simulink model "respiratory"  (R2020a)
settings: Solver=VariableStepAuto  StartTime=0.0  StopTime=17.0  RelTol=1e-3
settings Model: Creator=PrasunOrchi  LastModifiedBy=PrasunOrchi

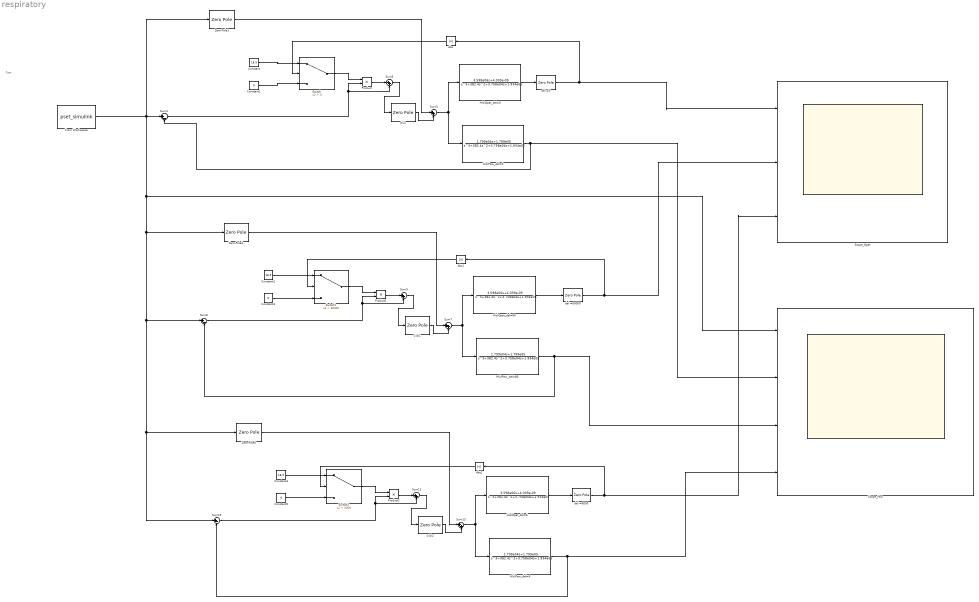
== system respiratory ==
  note: Pset
  Abs : Abs
  Abs1 : Abs
  Abs2 : Abs
  C(s) : ZeroPole  Zeros=[]  Poles=[0]  Gain=[0.4]
  C(s)1 : ZeroPole  Zeros=[]  Poles=[0]  Gain=[0.4]
  C(s)2 : ZeroPole  Zeros=[]  Poles=[0]  Gain=[0.4]
  Constant : Constant  Value=18.5
  Constant1 : Constant  Value=0
  Constant2 : Constant  Value=18.5
  Constant3 : Constant  Value=0
  Constant4 : Constant  Value=18.5
  Constant5 : Constant  Value=0
  From Workspace : FromWorkspace  VariableName=pset_simulink
  H(s)Paw_del=0 : TransferFcn  Numerator=[1.799e04 1.799e05]  Denominator=[1 382.4 3.758e04 1.934e05]
  H(s)Paw_del=6 : TransferFcn  Numerator=[1.799e04 1.799e05]  Denominator=[1 382.4 3.758e04 1.934e05]
  H(s)Paw_del=80 : TransferFcn  Numerator=[1.799e04 1.799e05]  Denominator=[1 382.4 3.758e04 1.934e05]
  H(s)Qpat_del=0 : TransferFcn  Numerator=[3.598e06 4.039e-09]  Denominator=[1 382.4 3.758e04 1.934e05]
  H(s)Qpat_del=6 : TransferFcn  Numerator=[3.598e06 4.039e-09]  Denominator=[1 382.4 3.758e04 1.934e05]
  H(s)Qpat_del=80 : TransferFcn  Numerator=[3.598e06 4.039e-09]  Denominator=[1 382.4 3.758e04 1.934e05]
  Product : Product
  Product1 : Product
  Product2 : Product
  Scope_Paw : Scope  NumInputPorts=4
  Scope_Qpat : Scope  NumInputPorts=3
  Sum10 : Sum  Inputs=|+-
  Sum{3,5,7,9,11,13} (6 alike) : Sum  Inputs=|++
  Sum4 : Sum  Inputs=|+-
  Sum8 : Sum  Inputs=|+-
  Switch : Switch  Criteria=u2 > Threshold
  Switch1 : Switch  Criteria=u2 > Threshold  Threshold=80000
  Switch2 : Switch  Criteria=u2 > Threshold  Threshold=6000
  Zero-Pole1 : ZeroPole  Zeros=[]  Poles=[]
  Zero-Pole3 : ZeroPole  Zeros=[]  Poles=[]
  Zero-Pole5 : ZeroPole  Zeros=[]  Poles=[]
  del =0 : ZeroPole  Zeros=[]  Poles=[]  Gain=[60]
  del =6000 : ZeroPole  Zeros=[]  Poles=[]  Gain=[60]
  del =80000 : ZeroPole  Zeros=[]  Poles=[]  Gain=[60]
  wires:
  Sum8/1 -> Sum9/2, Product1/2
  Sum9/1 -> C(s)1/1
  Sum5/1 -> C(s)/1
  Constant3/1 -> Switch1/3
  Switch/1 -> Product/1
  Constant1/1 -> Switch/3
  C(s)1/1 -> Sum7/2
  Constant2/1 -> Switch1/1
  Product/1 -> Sum5/1
  Constant/1 -> Switch/1
  H(s)Paw_del=6/1 -> Sum10/2, Scope_Paw/4
  Switch2/1 -> Product2/1
  Sum10/1 -> Sum11/2, Product2/2
  Sum3/1 -> H(s)Qpat_del=0/1, H(s)Paw_del=0/1
  Product2/1 -> Sum11/1
  H(s)Qpat_del=6/1 -> del =6000/1
  C(s)2/1 -> Sum13/2
  Sum13/1 -> H(s)Qpat_del=6/1, H(s)Paw_del=6/1
  Constant4/1 -> Switch2/1
  Product1/1 -> Sum9/1
  H(s)Qpat_del=80/1 -> del =80000/1
  Sum7/1 -> H(s)Qpat_del=80/1, H(s)Paw_del=80/1
  Constant5/1 -> Switch2/3
  Sum4/1 -> Sum5/2, Product/2
  Sum11/1 -> C(s)2/1
  H(s)Paw_del=80/1 -> Sum8/2, Scope_Paw/3
  Zero-Pole1/1 -> Sum3/1
  Zero-Pole3/1 -> Sum7/1
  Switch1/1 -> Product1/1
  C(s)/1 -> Sum3/2
  H(s)Paw_del=0/1 -> Scope_Paw/2, Sum4/2
  Zero-Pole5/1 -> Sum13/1
  H(s)Qpat_del=0/1 -> del =0/1
  del =0/1 -> Abs/1, Scope_Qpat/1
  del =80000/1 -> Abs1/1, Scope_Qpat/2
  From Workspace/1 -> Sum4/1, Zero-Pole1/1, Scope_Paw/1, Zero-Pole3/1, Zero-Pole5/1, Sum10/1, Sum8/1
  del =6000/1 -> Abs2/1, Scope_Qpat/3
  Abs/1 -> Switch/2
  Abs1/1 -> Switch1/2
  Abs2/1 -> Switch2/2
